simulink model "mosaic_2019b"  (R2024b)
settings: Solver=FixedStepDiscrete  StartTime=0.0  StopTime=50  RelTol=1e-3
undefined symbols (not defined in the file or in its folder): fspecial, gray
libraries: simulink x3, dspmtrx3 x2, visiontextngfix x2, visiongeotforms x2, visionanalysis x1, dspstat3 x1, visionsinks x1, visionsources x1
settings Model: Creator=FxMain  LastModifiedBy=Nick
settings SolverCC: AlgebraicLoopSolver=TrustRegion
settings DataIOCC: LimitDataPoints=on  SaveFormat=Array  SignalLoggingSaveFormat=ModelDataLogs  SaveOutput=off  SaveTime=off  ReturnWorkspaceOutputs=off
settings OptimizationCC: ExpressionDepthLimit=2147483647  LifeSpan=inf
settings DebuggingCC: UnderspecifiedInitializationDetection=Classic  MergeDetectMultiDrivingBlocksExec=none  SolverPrmCheckMsg=warning  FcnCallInpInsideContextMsg=warning  UnconnectedInputMsg=warning  UnconnectedOutputMsg=warning  UnconnectedLineMsg=warning  StateNameClashWarn=warning  SFUnexpectedBacktrackingDiag=warning  SFNoUnconditionalDefaultTransitionDiag=warning  SFExecutionAtInitializationDiag=none  ArithmeticOperatorsInVariantConditions=warning
settings HardwareCC: ProdBitPerPointer=32  ProdBitPerSizeT=32  ProdBitPerPtrDiffT=32  ProdLargestAtomicFloat=None  ProdIntDivRoundTo=Undefined  ProdEndianess=Unspecified  ProdWordSize=32  ProdHWDeviceType=32-bit Generic  TargetBitPerPointer=64  TargetBitPerSizeT=64  TargetBitPerPtrDiffT=64  TargetLongLongMode=on  TargetIntDivRoundTo=Zero  TargetEndianess=LittleEndian  TargetWordSize=64  TargetHWDeviceType=Generic->MATLAB Host Computer  ProdEqTarget=off
settings ModelReferenceCC: EnableRefExpFcnMdlSchedulingChecks=on  PropagateSignalLabelsOutOfModel=off
settings SFSimCC: SimUseLocalCustomCode=off  CustomCodeUndefinedFunction=UseInterfaceOnly
settings RTWCC: RTWUseLocalCustomCode=off  GPUComputeCapability=3.5
settings CodeAppCC: StateflowObjectComments=on
settings GRTTargetCC: TargetLangStandard=C89/C90 (ANSI)  CombineOutputUpdateFcns=off  GRTInterface=on
settings ConfigComp: CovMetricSettings=dw  CovSaveCumulativeToWorkspaceVar=on  CovSaveSingleToWorkspaceVar=on

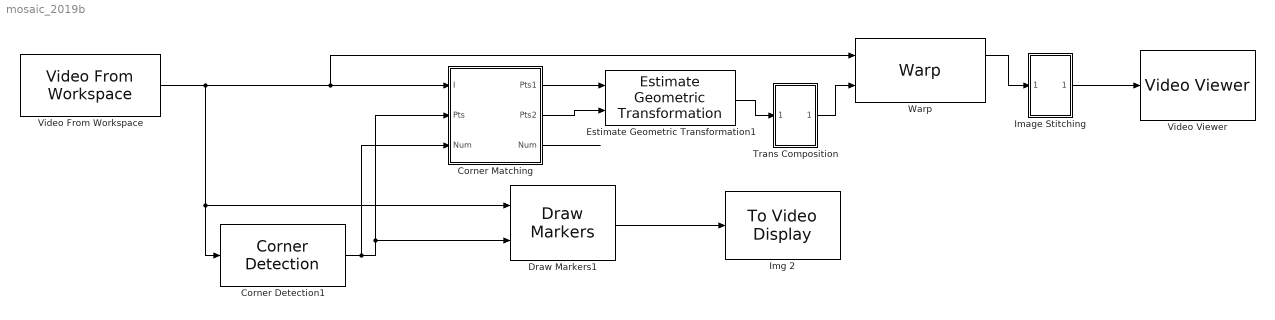
== system mosaic_2019b ==
  Corner Detection1 : visionanalysis/Corner Detection  method=Harris corner detection (Harris & Stephens)  factor=0.04  filter=fspecial('gaussian', [1 5], 1.5)  thrInten=0.1  thrAngle=157.5  output=Obsolete9b  outputInUse=Corner location  maxNum=200  thrMetric=0.0005  neighborSize=[11 11]  isOutVarDim=on  roundingMode=Floor  overflowMode=off  firstCoeffMode=Specify word length  firstCoeffWordLength=16  firstCoeffFracLength=16  prodOutputMode=Binary point scaling  prodOutputWordLength=32  prodOutputFracLength=0  accumMode=Binary point scaling  accumWordLength=32  accumFracLength=0  memoryMode=Binary point scaling  memoryWordLength=32  memoryFracLength=0
  Corner Matching : Subsystem  mask(Corner Matching){winLen=9, maxNum=75, threshold=81}
      mask prompts: winLen "Block size used in corner matching:"; maxNum "Maximum number of points:"; threshold "Maximum feature difference for matching points:"
      mask help: Find out matching corners in the current and previous video frames.
  Draw Markers1 : visiontextngfix/Draw Markers  shape=Circle  size=3  fill=off  fillClrSource=Specify via dialog  display=Black  intensity=200  color=[200 255 100]  opacity=0.6  viewport=Entire image  antialiasing=off  inType=Obsolete  imagePorts=One multidimensional signal  roundingMode=Floor  overflowMode=off  memoryMode=Specify word length  memoryWordLength=16  memoryFracLength=15  prodOutputMode=Binary point scaling  prodOutputWordLength=32  prodOutputFracLength=14
  Estimate Geometric Transformation1 : visiongeotforms/Estimate Geometric Transformation  tformType=Affine  isRandomSampling=on  algMethod=Random Sample Consensus (RANSAC)  distanceAlg=2.5  distanceGeo=2.5  numMethod=Specified value  sampleNum=500  desiredConfidence=99  maxSampleNum=1000  isStopSampling=off  percentStop=75  isRefineTForm=off  isReleaseMode=on  isOutputInlier=off  outDT4IntInput=Obsolete10a  outDT4IntInputActive=Single  isVarSizeAllowed=on
  Image Stitching : Subsystem
  Img 2 : visionsinks/To Video Display  windowSizeMode=True size (1:1)  openAtMdlStart=on  fullScreen=off  videoWindowX=94  videoWindowY=125  saveWindowSize=off  videoWindowWidth=640  videoWindowHeight=480  inputColorFormat=RGB  inputType=Obsolete  imagePorts=One multidimensional signal  OutputDevice=On-screen video monitor  dataOrg=Column-major  isWindowOpen=off
  Trans Composition : Subsystem
  Video From Workspace : visionsources/Video From Workspace  signal=vid1  Ts=1  finalout=Obsolete  finaloutActive=Cyclic repetition  imagePorts=One multidimensional signal  OutPortLabels=R|G|B
  Video Viewer : VideoViewer  colormapValue=gray(256)  FigPos=[600 444 721 182]  trueSizedOnce=on
  Warp : visiongeotforms/Warp  TransformMatrixSource=Input port  TransformMatrix=eye( 3 )  InterpolationMethod=Bilinear  BackgroundFillValue=0  OutputImagePositionSource=Same as input image  OutputImagePosition=[ 1, 1, 512, 512 ]  ROIInputPort=off  ROIValidityOutputPort=on  SimulateUsing=Interpreted execution
  wires:
  Draw Markers1/1 -> Img 2/1
  Corner Matching/1(Pts1) -> Estimate Geometric Transformation1/1
  Corner Matching/2(Pts2) -> Estimate Geometric Transformation1/2
  Corner Detection1/1 -> Corner Matching/3(Num), Draw Markers1/2, Corner Matching/2(Pts)
  Estimate Geometric Transformation1/1 -> Trans Composition/1(In1)
  Corner Matching/3("Num ") -> ?
  Video From Workspace/1 -> Warp/1, Corner Matching/1(I), Corner Detection1/1, Draw Markers1/1
  Trans Composition/1(Out1) -> Warp/2
  Warp/1 -> Image Stitching/1(In1)
  Image Stitching/1(Out1) -> Video Viewer/1

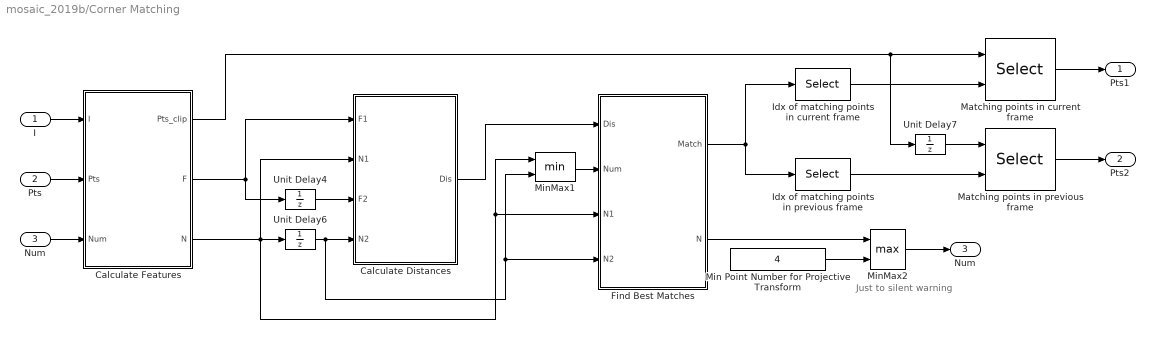
== system mosaic_2019b/Corner Matching ==
  note: Just to
      | silent warning
  I : Inport
  Pts : Inport  Port=2
  Num : Inport  Port=3
  Calculate Distances : Subsystem  TreatAsAtomicUnit=on  mask{maxNum=maxNum}
      mask prompts: maxNum "Maximum data number:"
      settings: AttributesFormatString=between features.
  Calculate Features : Subsystem  TreatAsAtomicUnit=on  mask{winLen=winLen, maxNum=maxNum}
      mask prompts: winLen "Neighborhood size:"; maxNum "Maximum number of features:"
  Find Best Matches : Subsystem  TreatAsAtomicUnit=on  mask{maxNum=maxNum, threshold=threshold}
      mask prompts: maxNum "Maximum data number:"
      settings: AttributesFormatString=between the features\nin the current and previous frames
  Idx of matching points in current frame : Selector  NumberOfDimensions=2  IndexMode=Zero-based  InputPortWidth=2  IndexOptions=Index vector (dialog),Select all  Indices=0,1  OutputSizes=1,1
  Idx of matching points in previous frame : Selector  NumberOfDimensions=2  IndexMode=Zero-based  InputPortWidth=2  IndexOptions=Index vector (dialog),Select all  Indices=1,1  OutputSizes=1,1
  Matching points in current frame : Selector  NumberOfDimensions=2  IndexMode=Zero-based  InputPortWidth=2  IndexOptions=Select all,Index vector (port)  Indices=0,1  OutputSizes=1,1
  Matching points in previous frame : Selector  NumberOfDimensions=2  IndexMode=Zero-based  InputPortWidth=2  IndexOptions=Select all,Index vector (port)  Indices=0,1  OutputSizes=1,1
  Min Point Number for Projective Transform : Constant  Value=4  OutDataTypeStr=Inherit: Inherit via back propagation
  MinMax1 : MinMax  Inputs=2
  MinMax2 : MinMax  Function=max  Inputs=2  OutDataTypeStr=Inherit: Inherit via back propagation
  Unit Delay4 : UnitDelay  SampleTime=-1
  Unit Delay6 : UnitDelay  SampleTime=-1
  Unit Delay7 : UnitDelay  SampleTime=-1
  Pts1 : Outport
  Pts2 : Outport  Port=2
  "Num " : Outport  Port=3
  wires:
  Calculate Features/2(F) -> Calculate Distances/1(F1), Unit Delay4/1
  Calculate Features/3(N) -> Calculate Distances/2(N1), Unit Delay6/1, MinMax1/1, Find Best Matches/3(N1)
  Calculate Features/1(Pts_clip) -> Unit Delay7/1, Matching points in current frame/1
  Num/1 -> Calculate Features/3(Num)
  Unit Delay6/1 -> Calculate Distances/4(N2), MinMax1/2, Find Best Matches/4(N2)
  Unit Delay4/1 -> Calculate Distances/3(F2)
  Matching points in previous frame/1 -> Pts2/1
  Matching points in current frame/1 -> Pts1/1
  Unit Delay7/1 -> Matching points in previous frame/1
  Idx of matching points in current frame/1 -> Matching points in current frame/2
  Idx of matching points in previous frame/1 -> Matching points in previous frame/2
  Find Best Matches/1(Match) -> Idx of matching points in previous frame/1, Idx of matching points in current frame/1
  Calculate Distances/1(Dis) -> Find Best Matches/1(Dis)
  I/1 -> Calculate Features/1(I)
  Pts/1 -> Calculate Features/2(Pts)
  Min Point Number for Projective Transform/1 -> MinMax2/2
  Find Best Matches/2(N) -> MinMax2/1
  MinMax2/1 -> "Num "/1
  MinMax1/1 -> Find Best Matches/2(Num)

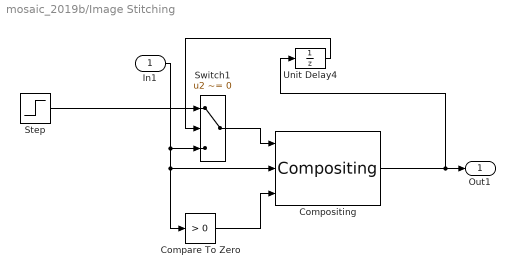
== system mosaic_2019b/Image Stitching ==
  In1 : Inport
  Compare To Zero : simulink/Logic and Bit Operations/Compare To Zero  relop=>  OutDataTypeStr=boolean  ZeroCross=off
  Compositing : visiontextngfix/Compositing  operation=Binary mask  bFacSrc=Specify via dialog  bFactor=0.5  mFacSrc=Input port  mFactor=1  source=Specify via dialog  coordinates=[0 0]  roundingMode=Floor  overflowMode=off  prodOutputMode=Binary point scaling  prodOutputWordLength=32  prodOutputFracLength=10
  Step : Step  Time=2  SampleTime=0
  Switch1 : Switch  Criteria=u2 ~= 0  ZeroCross=off  SaturateOnIntegerOverflow=off
  Unit Delay4 : UnitDelay  SampleTime=-1
  Out1 : Outport
  wires:
  Step/1 -> Switch1/2
  Switch1/1 -> Compositing/1
  Unit Delay4/1 -> Switch1/1
  In1/1 -> Switch1/3, Compare To Zero/1, Compositing/2
  Compositing/1 -> Out1/1, Unit Delay4/1
  Compare To Zero/1 -> Compositing/3

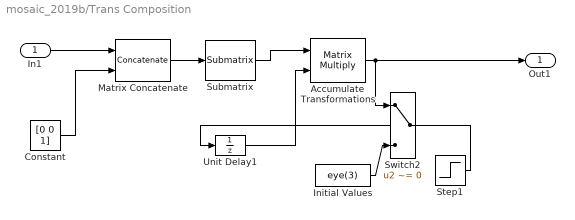
== system mosaic_2019b/Trans Composition ==
  In1 : Inport
  Accumulate Transformations : Product  Multiplication=Matrix(*)  InputSameDT=on  RndMeth=Zero
  Constant : Constant  Value=[0 0 1]  VectorParams1D=off
      settings: SamplingMode=Frame based
  Initial Values : Constant  Value=eye(3)  OutDataTypeStr=Inherit: Inherit via back propagation  SampleTime=-1
  Matrix Concatenate : Concatenate  Mode=Multidimensional array
  Step1 : Step  Time=2  SampleTime=0
  Submatrix : dspmtrx3/Submatrix  RowSpan=Range of rows  RowStartMode=First  RowStartIndex=1  RowEndMode=Index  RowEndIndex=3  ColSpan=All columns  ColStartMode=First  ColStartIndex=1  ColEndMode=Last  ColEndIndex=1
  Switch2 : Switch  Criteria=u2 ~= 0  ZeroCross=off  SaturateOnIntegerOverflow=off
  Unit Delay1 : UnitDelay  SampleTime=-1
  Out1 : Outport
  wires:
  Accumulate Transformations/1 -> Out1/1, Switch2/1
  Unit Delay1/1 -> Accumulate Transformations/2
  Switch2/1 -> Unit Delay1/1
  Initial Values/1 -> Switch2/3
  Step1/1 -> Switch2/2
  In1/1 -> Matrix Concatenate/1
  Constant/1 -> Matrix Concatenate/2
  Submatrix/1 -> Accumulate Transformations/1
  Matrix Concatenate/1 -> Submatrix/1

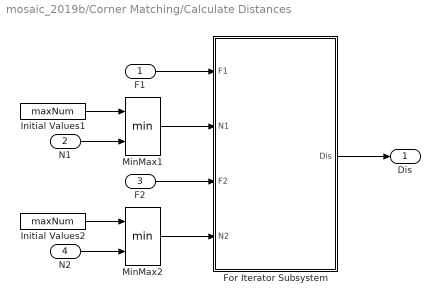
== system mosaic_2019b/Corner Matching/Calculate Distances ==
  F1 : Inport
  N1 : Inport  Port=2
  F2 : Inport  Port=3
  N2 : Inport  Port=4
  For Iterator Subsystem : Subsystem  TreatAsAtomicUnit=on
  Initial Values1 : Constant  Value=maxNum  OutDataTypeStr=Inherit: Inherit via back propagation  SampleTime=-1
  Initial Values2 : Constant  Value=maxNum  OutDataTypeStr=Inherit: Inherit via back propagation  SampleTime=-1
  MinMax1 : MinMax  Inputs=2
  MinMax2 : MinMax  Inputs=2
  Dis : Outport
  wires:
  MinMax2/1 -> For Iterator Subsystem/4(N2)
  F2/1 -> For Iterator Subsystem/3(F2)
  MinMax1/1 -> For Iterator Subsystem/2(N1)
  F1/1 -> For Iterator Subsystem/1(F1)
  For Iterator Subsystem/1(Dis) -> Dis/1
  N2/1 -> MinMax2/2
  Initial Values2/1 -> MinMax2/1
  N1/1 -> MinMax1/2
  Initial Values1/1 -> MinMax1/1

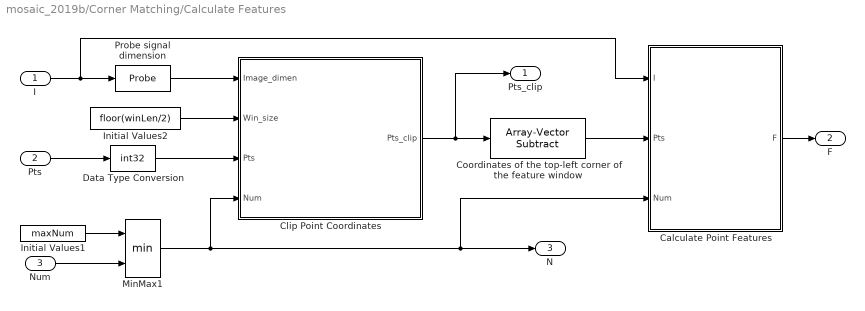
== system mosaic_2019b/Corner Matching/Calculate Features ==
  I : Inport
  Pts : Inport  Port=2
  Num : Inport  Port=3
  Calculate Point Features : Subsystem
  Clip Point Coordinates : Subsystem
  Coordinates of the top-left corner of the feature window : dspmtrx3/Array-Vector Subtract  Dimension=1  V_Source=Dialog parameter  V_VectFromMask=floor([winLen; winLen] / 2)  prodOutputSignedness=Auto  roundingMode=Floor  overflowMode=off  firstCoeffSignedness=Auto  firstCoeffDataTypeStr=Inherit: Same word length as input  firstCoeffMin=[]  firstCoeffMax=[]  firstCoeffLastDataTypeStr=Inherit: Same word length as input  accumSignedness=Auto  outputSignedness=Auto  outputMin=[]  outputMax=[]
  Data Type Conversion : DataTypeConversion  OutDataTypeStr=int32  SaturateOnIntegerOverflow=off  RndMeth=Floor
  Initial Values1 : Constant  Value=maxNum  OutDataTypeStr=Inherit: Inherit via back propagation  SampleTime=-1
  Initial Values2 : Constant  Value=floor(winLen/2)  OutDataTypeStr=Inherit: Inherit via back propagation  SampleTime=-1
  MinMax1 : MinMax  Inputs=2
  Probe signal dimension : Probe  ProbeWidth=off  ProbeSampleTime=off  ProbeComplexSignal=off  ProbeSignalDimensions=on  ProbeDimensionsDataType=int32
  Pts_clip : Outport
  F : Outport  Port=2
  N : Outport  Port=3
  wires:
  Data Type Conversion/1 -> Clip Point Coordinates/3(Pts)
  MinMax1/1 -> N/1, Calculate Point Features/3(Num), Clip Point Coordinates/4(Num)
  Coordinates of the top-left corner of the feature window/1 -> Calculate Point Features/2(Pts)
  Clip Point Coordinates/1(Pts_clip) -> Coordinates of the top-left corner of the feature window/1, Pts_clip/1
  Pts/1 -> Data Type Conversion/1
  Initial Values2/1 -> Clip Point Coordinates/2(Win_size)
  Probe signal dimension/1 -> Clip Point Coordinates/1(Image_dimen)
  I/1 -> Calculate Point Features/1(I), Probe signal dimension/1
  Initial Values1/1 -> MinMax1/1
  Num/1 -> MinMax1/2
  Calculate Point Features/1(F) -> F/1

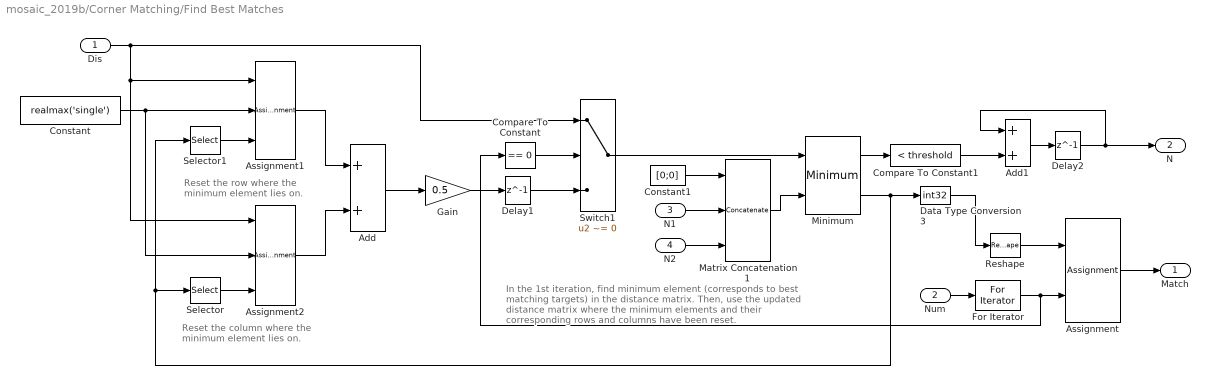
== system mosaic_2019b/Corner Matching/Find Best Matches ==
  note: In the 1st iteration, find minimum element (corresponds to
      | best matching targets) in the distance matrix. Then, use the
      | updated distance matrix where the minimum elements and
      | their  corresponding rows and columns have been reset.
  note: Reset the column where the
      | minimum element lies on.
  note: Reset the row where the
      | minimum element lies on.
  Dis : Inport
  Num : Inport  Port=2
  N1 : Inport  Port=3
  N2 : Inport  Port=4
  Add : Sum
  Add1 : Sum  OutDataTypeStr=int32
  Assignment : Assignment  NumberOfDimensions=2  IndexMode=Zero-based  OutputInitialize=Specify size for each dimension in table  IndexOptions=Assign all,Index vector (port)  Indices=-1,-1  OutputSizes=2,maxNum
  Assignment1 : Assignment  NumberOfDimensions=2  IndexMode=Zero-based  IndexOptions=Index vector (port),Assign all  Indices=1,-1  OutputSizes=1,1
  Assignment2 : Assignment  NumberOfDimensions=2  IndexMode=Zero-based  IndexOptions=Assign all,Index vector (port)  Indices=-1,-1  OutputSizes=1,1
  Compare To Constant : simulink/Logic and Bit Operations/Compare To Constant  relop===  const=0  OutDataTypeStr=boolean  ZeroCross=off
  Compare To Constant1 : simulink/Logic and Bit Operations/Compare To Constant  relop=<  const=threshold  OutDataTypeStr=uint8  ZeroCross=off
  Constant : Constant  Value=realmax('single')  VectorParams1D=off  OutDataTypeStr=Inherit: Inherit via back propagation
  Constant1 : Constant  Value=[0;0]  VectorParams1D=off  OutDataTypeStr=Inherit: Inherit via back propagation
  Data Type Conversion3 : DataTypeConversion  OutDataTypeStr=int32
  Delay1 : Delay  DelayLength=1  InitialCondition=0
  Delay2 : Delay  DelayLength=1  InitialCondition=0
  For Iterator : ForIterator  ResetStates=reset  IterationSource=external  IterationLimit=expLaneNum  IndexMode=Zero-based
  Gain : Gain  Gain=0.5
  Matrix Concatenation1 : Concatenate  NumInputs=3  Mode=Multidimensional array
  Minimum : dspstat3/Minimum  operation=minimum  fcn=Value and Index  indexBase=Zero  operateOver=Entire input  Dimension=1  InputProcessing=Columns as channels (frame based)  reset=None  roiEnable=on  roiType=Rectangles  roiPortion=Entire ROI  roiOutput=Individual statistics for each ROI  roiFlag=off  roundingMode=Floor  overflowMode=off
  Reshape : Reshape  OutputDimensionality=Column vector (2-D)
  Selector : Selector  IndexMode=Zero-based  InputPortWidth=2  IndexOptions=Index vector (dialog)  Indices=1  OutputSizes=1
  Selector1 : Selector  IndexMode=Zero-based  InputPortWidth=2  IndexOptions=Index vector (dialog)  Indices=0  OutputSizes=1
  Switch1 : Switch  Criteria=u2 ~= 0  SaturateOnIntegerOverflow=off  InputSameDT=off
  Match : Outport
  N : Outport  Port=2
  wires:
  Gain/1 -> Delay1/1
  Minimum/1 -> Compare To Constant1/1
  Compare To Constant1/1 -> Add1/2
  Delay2/1 -> Add1/1, N/1
  Add1/1 -> Delay2/1
  Num/1 -> For Iterator/1
  Data Type Conversion3/1 -> Reshape/1
  Compare To Constant/1 -> Switch1/2
  For Iterator/1 -> Compare To Constant/1, Assignment/2
  Switch1/1 -> Minimum/1
  Dis/1 -> Switch1/1, Assignment2/1, Assignment1/1
  Delay1/1 -> Switch1/3
  Assignment/1 -> Match/1
  Selector1/1 -> Assignment1/3
  Assignment1/1 -> Add/1
  Assignment2/1 -> Add/2
  Add/1 -> Gain/1
  Minimum/2 -> Data Type Conversion3/1, Selector/1, Selector1/1
  Constant/1 -> Assignment1/2, Assignment2/2
  Selector/1 -> Assignment2/3
  Constant1/1 -> Matrix Concatenation1/1
  N1/1 -> Matrix Concatenation1/2
  N2/1 -> Matrix Concatenation1/3
  Matrix Concatenation1/1 -> Minimum/2
  Reshape/1 -> Assignment/1

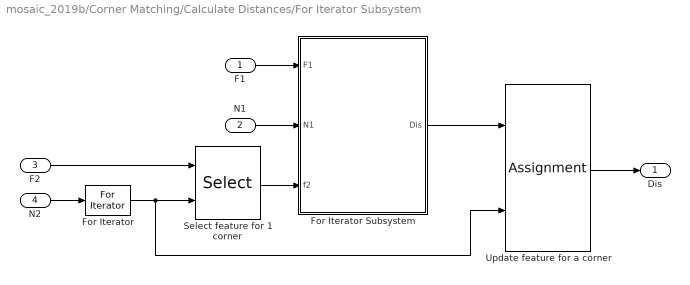
== system mosaic_2019b/Corner Matching/Calculate Distances/For Iterator Subsystem ==
  F1 : Inport
  N1 : Inport  Port=2
  F2 : Inport  Port=3
  N2 : Inport  Port=4
  For Iterator : ForIterator  IterationSource=external  IndexMode=Zero-based
  For Iterator Subsystem : Subsystem  TreatAsAtomicUnit=on
  Select feature for 1 corner : Selector  NumberOfDimensions=2  IndexMode=Zero-based  InputPortWidth=2  IndexOptions=Select all,Index vector (port)  Indices=0,1  OutputSizes=1,1
  Update feature for a corner : Assignment  NumberOfDimensions=2  IndexMode=Zero-based  OutputInitialize=Specify size for each dimension in table  IndexOptions=Assign all,Index vector (port)  Indices=1,1  OutputSizes=maxNum,maxNum
  Dis : Outport
  wires:
  Update feature for a corner/1 -> Dis/1
  N1/1 -> For Iterator Subsystem/2(N1)
  F1/1 -> For Iterator Subsystem/1(F1)
  Select feature for 1 corner/1 -> For Iterator Subsystem/3(f2)
  F2/1 -> Select feature for 1 corner/1
  For Iterator/1 -> Select feature for 1 corner/2, Update feature for a corner/2
  N2/1 -> For Iterator/1
  For Iterator Subsystem/1(Dis) -> Update feature for a corner/1

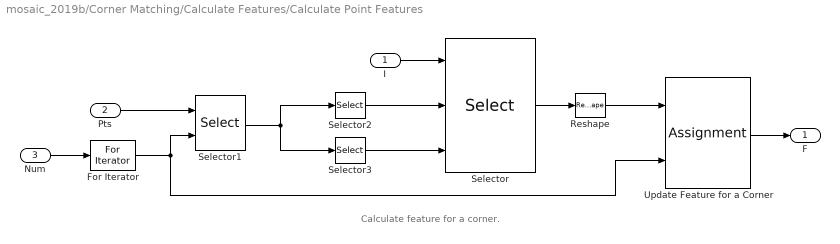
== system mosaic_2019b/Corner Matching/Calculate Features/Calculate Point Features ==
  note: Calculate feature for a corner.
  I : Inport
  Pts : Inport  Port=2
  Num : Inport  Port=3
  For Iterator : ForIterator  IterationSource=external  IndexMode=Zero-based
  Reshape : Reshape  OutputDimensionality=Column vector (2-D)
  Selector : Selector  NumberOfDimensions=2  IndexMode=Zero-based  InputPortWidth=3  IndexOptions=Starting index (port),Starting index (port)  Indices=[1 3],1  OutputSizes=winLen,winLen
  Selector1 : Selector  NumberOfDimensions=2  IndexMode=Zero-based  InputPortWidth=3  IndexOptions=Select all,Index vector (port)  Indices=[1 3],1  OutputSizes=9,9
  Selector2 : Selector  IndexMode=Zero-based  InputPortWidth=2  IndexOptions=Index vector (dialog)  Indices=0  OutputSizes=9
  Selector3 : Selector  IndexMode=Zero-based  InputPortWidth=2  IndexOptions=Index vector (dialog)  Indices=1  OutputSizes=9
  Update Feature for a Corner : Assignment  NumberOfDimensions=2  IndexMode=Zero-based  OutputInitialize=Specify size for each dimension in table  IndexOptions=Assign all,Index vector (port)  Indices=1,1  OutputSizes=winLen^2,maxNum
  F : Outport
  wires:
  Selector3/1 -> Selector/3
  Selector2/1 -> Selector/2
  Num/1 -> For Iterator/1
  Update Feature for a Corner/1 -> F/1
  Pts/1 -> Selector1/1
  I/1 -> Selector/1
  Reshape/1 -> Update Feature for a Corner/1
  Selector/1 -> Reshape/1
  Selector1/1 -> Selector2/1, Selector3/1
  For Iterator/1 -> Update Feature for a Corner/2, Selector1/2

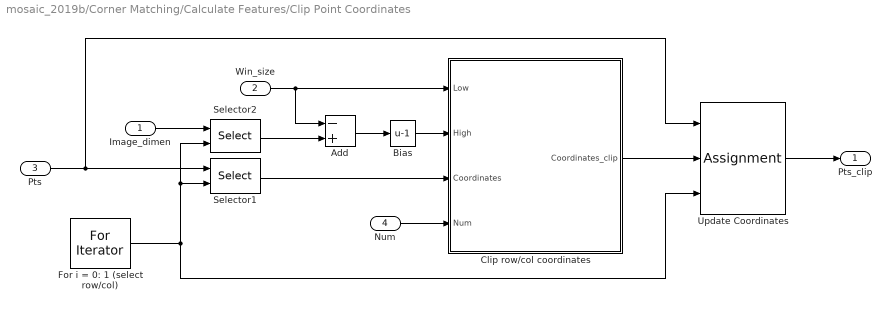
== system mosaic_2019b/Corner Matching/Calculate Features/Clip Point Coordinates ==
  Image_dimen : Inport
  Win_size : Inport  Port=2
  Pts : Inport  Port=3
  Num : Inport  Port=4
  Add : Sum  Inputs=-+
  Bias : Bias  Bias=-1  SaturateOnIntegerOverflow=off
  Clip row/col coordinates : Subsystem
  For i = 0: 1 (select row/col) : ForIterator  IterationLimit=2  IndexMode=Zero-based
  Selector1 : Selector  NumberOfDimensions=2  IndexMode=Zero-based  InputPortWidth=3  IndexOptions=Index vector (port),Select all  Indices=[1 3],1  OutputSizes=9,9
  Selector2 : Selector  IndexMode=Zero-based  InputPortWidth=2  IndexOptions=Index vector (port)  Indices=[1 3]  OutputSizes=9
  Update Coordinates : Assignment  NumberOfDimensions=2  IndexMode=Zero-based  IndexOptions=Index vector (port),Assign all  Indices=1,1  OutputSizes=81,50
  Pts_clip : Outport
  wires:
  Selector2/1 -> Add/2
  For i = 0: 1 (select row/col)/1 -> Selector1/2, Selector2/2, Update Coordinates/3
  Clip row/col coordinates/1(Coordinates_clip) -> Update Coordinates/2
  Bias/1 -> Clip row/col coordinates/2(High)
  Update Coordinates/1 -> Pts_clip/1
  Num/1 -> Clip row/col coordinates/4(Num)
  Selector1/1 -> Clip row/col coordinates/3(Coordinates)
  Win_size/1 -> Add/1, Clip row/col coordinates/1(Low)
  Add/1 -> Bias/1
  Image_dimen/1 -> Selector2/1
  Pts/1 -> Update Coordinates/1, Selector1/1

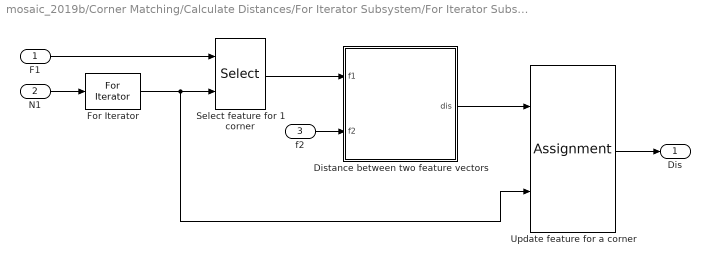
== system mosaic_2019b/Corner Matching/Calculate Distances/For Iterator Subsystem/For Iterator Subsystem ==
  F1 : Inport
  N1 : Inport  Port=2
  f2 : Inport  Port=3
  Distance between two feature vectors : Subsystem
  For Iterator : ForIterator  IterationSource=external  IndexMode=Zero-based
  Select feature for 1 corner : Selector  NumberOfDimensions=2  IndexMode=Zero-based  InputPortWidth=2  IndexOptions=Select all,Index vector (port)  Indices=0,1  OutputSizes=1,1
  Update feature for a corner : Assignment  NumberOfDimensions=2  IndexMode=Zero-based  OutputInitialize=Specify size for each dimension in table  IndexOptions=Index vector (port),Assign all  Indices=1,1  OutputSizes=maxNum,1
  Dis : Outport
  wires:
  Select feature for 1 corner/1 -> Distance between two feature vectors/1(f1)
  f2/1 -> Distance between two feature vectors/2(f2)
  Update feature for a corner/1 -> Dis/1
  F1/1 -> Select feature for 1 corner/1
  For Iterator/1 -> Select feature for 1 corner/2, Update feature for a corner/2
  N1/1 -> For Iterator/1
  Distance between two feature vectors/1(dis) -> Update feature for a corner/1

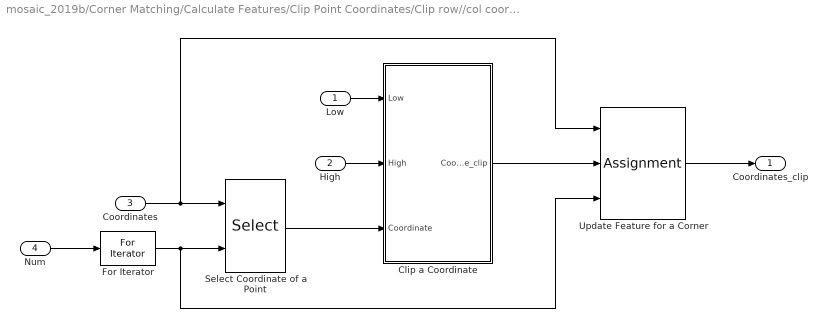
== system mosaic_2019b/Corner Matching/Calculate Features/Clip Point Coordinates/Clip row//col coordinates ==
  Low : Inport
  High : Inport  Port=2
  Coordinates : Inport  Port=3
  Num : Inport  Port=4
  Clip a Coordinate : Subsystem
  For Iterator : ForIterator  IterationSource=external  IterationLimit=2  IndexMode=Zero-based
  Select Coordinate of a Point : Selector  NumberOfDimensions=2  IndexMode=Zero-based  InputPortWidth=3  IndexOptions=Select all,Index vector (port)  Indices=[1 3],1  OutputSizes=9,1
  Update Feature for a Corner : Assignment  NumberOfDimensions=2  IndexMode=Zero-based  IndexOptions=Assign all,Index vector (port)  Indices=1,1  OutputSizes=81,50
  Coordinates_clip : Outport
  wires:
  Clip a Coordinate/1(Coordinate_clip) -> Update Feature for a Corner/2
  Update Feature for a Corner/1 -> Coordinates_clip/1
  High/1 -> Clip a Coordinate/2(High)
  Low/1 -> Clip a Coordinate/1(Low)
  Select Coordinate of a Point/1 -> Clip a Coordinate/3(Coordinate)
  Num/1 -> For Iterator/1
  Coordinates/1 -> Update Feature for a Corner/1, Select Coordinate of a Point/1
  For Iterator/1 -> Select Coordinate of a Point/2, Update Feature for a Corner/3

== system mosaic_2019b/Corner Matching/Calculate Distances/For Iterator Subsystem/For Iterator Subsystem/Distance between two feature vectors ==
  f1 : Inport
  f2 : Inport  Port=2
  Abs : Abs  SaturateOnIntegerOverflow=off
  Add : Sum  Inputs=+-
  Sum of Elements : Sum  Inputs=+
  dis : Outport
  wires:
  Sum of Elements/1 -> dis/1
  Abs/1 -> Sum of Elements/1
  Add/1 -> Abs/1
  f2/1 -> Add/2
  f1/1 -> Add/1

== system mosaic_2019b/Corner Matching/Calculate Features/Clip Point Coordinates/Clip row//col coordinates/Clip a Coordinate ==
  Low : Inport
  High : Inport  Port=2
  Coordinate : Inport  Port=3
  MinMax1 : MinMax  Function=max  Inputs=2
  MinMax2 : MinMax  Inputs=2
  Coordinate_clip : Outport
  wires:
  MinMax2/1 -> Coordinate_clip/1
  High/1 -> MinMax2/2
  MinMax1/1 -> MinMax2/1
  Low/1 -> MinMax1/2
  Coordinate/1 -> MinMax1/1
